simulink model "MotorModel"  (R2021b)
settings: Solver=ode23tb  StartTime=0.0  StopTime=10  RelTol=1e-6
undefined symbols (not defined in the file): sigbuilder_block
libraries: slpidlib x4, aerolibanimutils x1
settings Model: Creator=user  LastModifiedBy=user

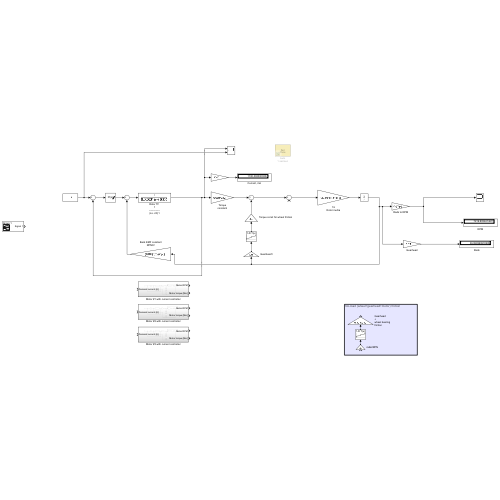
[thumbnail: Simulink's stored preview of the top-level diagram]
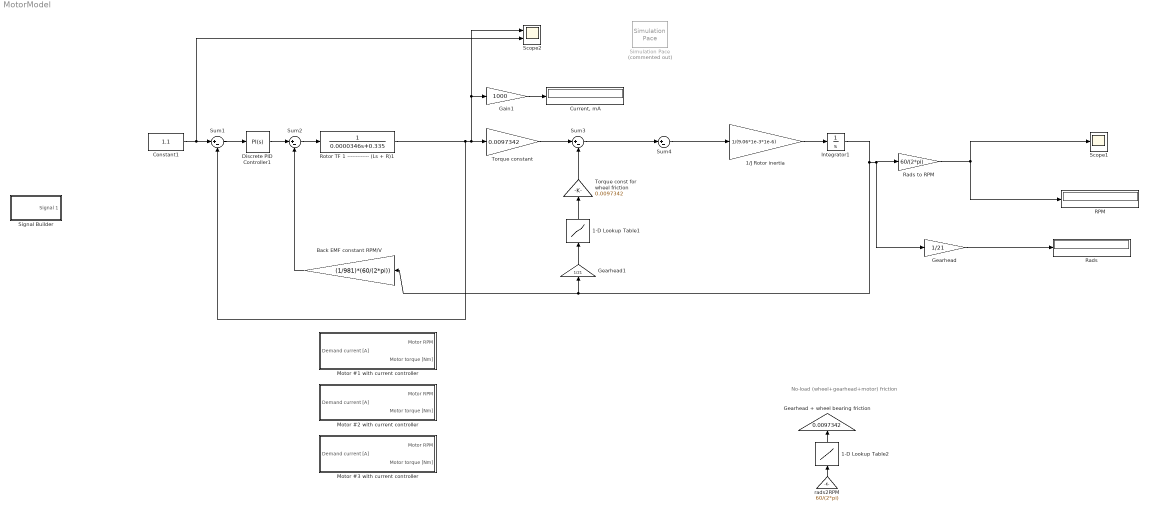
== system MotorModel ==
  note: No-load (wheel+gearhead+motor) friction
  1-D Lookup Table1 : Lookup_n-D  NumberOfTableDimensions=1  BreakpointsForDimension1=[-38 -37 -0.01 0.01 37 38]  Table=[-2 -1.1 -0.5 0.5 1.1 2]  InternalRulePriority=Speed  RndMeth=Simplest  InputSameDT=on
  1-D Lookup Table2 : Lookup_n-D  NumberOfTableDimensions=1  BreakpointsForDimension1=[-10658 -10600 -0.01 0.01 10600 10658]  Table=[-0.5 -0.25 -0.115 0.115 0.25 0.5]  InternalRulePriority=Speed  RndMeth=Simplest  InputSameDT=on
  1/J Rotor inertia : Gain  Gain=1/(9.06*1e-3*1e-6)
  Back EMF constant RPM/V : Gain  Gain=(1/981)*(60/(2*pi))
  Constant1 : Constant  Value=1.1
  "Current, mA" : Display
  Discrete PID Controller1 : slpidlib/PID Controller  Controller=PI  Form=Parallel  TimeDomain=Continuous-time  UseExternalTs=off  SampleTime=1e-6  IntegratorMethod=Forward Euler  FilterMethod=Forward Euler  ControllerParametersSource=internal  P=291  I=291/(1e-6*237)  D=0  UseFilter=on  N=100  TunerSelectOption=Transfer Function Based (PID Tuner App)  InitialConditionSource=internal  InitialConditionForIntegrator=0  InitialConditionForFilter=0  DifferentiatorICPrevScaledInput=0  ExternalReset=none  TrackingMode=off  Kt=1  LimitOutput=on  SatLimitsSource=internal  UpperSaturationLimit=12  LowerSaturationLimit=-12  LinearizeAsGain=off  AntiWindupMode=none  Kb=1  POutMin=[]  POutMax=[]  IOutMin=[]  IOutMax=[]  DOutMin=[]  DOutMax=[]  NOutMin=[]  NOutMax=[]  SumOutMin=[]  SumOutMax=[]  SaturationOutMin=[]  SaturationOutMax=[]  PParamMin=[]  PParamMax=[]  IParamMin=[]  IParamMax=[]  DParamMin=[]  DParamMax=[]  NParamMin=[]  NParamMax=[]  KbParamMin=[]  KbParamMax=[]  KtParamMin=[]  KtParamMax=[]  KbOutMin=[]  KbOutMax=[]  KtOutMin=[]  KtOutMax=[]  IntegratorOutMin=[]  IntegratorOutMax=[]  FilterOutMin=[]  FilterOutMax=[]  SumI1OutMin=[]  SumI1OutMax=[]  SumI2OutMin=[]  SumI2OutMax=[]  SumI3OutMin=[]  SumI3OutMax=[]  SumI4OutMin=[]  SumI4OutMax=[]  SumDOutMin=[]  SumDOutMax=[]  DifferentiatorOutMin=[]  DifferentiatorOutMax=[]  FilterDiffOutCoefMin=[]  FilterDiffOutCoefMax=[]  ReciprocalOutMin=[]  ReciprocalOutMax=[]  SumDenOutMin=[]  SumDenOutMax=[]  SumNumOutMin=[]  SumNumOutMax=[]  DivideOutMin=[]  DivideOutMax=[]  UdiffTsProdOutMin=[]  UdiffTsProdOutMax=[]  NTsProdOutMin=[]  NTsProdOutMax=[]  UintegralTsProdOutMin=[]  UintegralTsProdOutMax=[]  UngainTsProdOutMin=[]  UngainTsProdOutMax=[]  IntegratorContinuousStateAttributes=''  IntegratorStateMustResolveToSignalObject=off  IntegratorRTWStateStorageClass=Auto  FilterContinuousStateAttributes=''  FilterStateMustResolveToSignalObject=off  FilterRTWStateStorageClass=Auto  ParallelPVariant=InternalParameters  IdealPVariant=Disabled  IVariant=InternalParameters  DVariant=Disabled  IntegratorVariant=Continuous  SatVariant=Enabled  AWVariant=Passthrough  PCopyVariant=Disabled  TRVariant=Disabled  FdbkBlocksVariant=Forward  IdealPFdbkVariant=Disabled  SatFdbkVariant=Disabled  DerivativeFilterVariant=Disabled  NVariant=Disabled  NCopyVariant=Disabled_SignalSpec  FilterICVariant=Disabled  IntegratorICVariant=InternalICs  ExternalResetVariant=Disabled  TRSumVariant=Passthrough  SumFdbkVariant=Disabled  SumVariant=Sum_PI  TsampFilterVariant=InternalTs  TsampNgainVariant=Passthrough  TsampIntegralVariant=Passthrough  ExternalSaturationOutDataTypeStr=Inherit: Same as second input
  Gain1 : Gain  Gain=1000
  Gearhead : Gain  Gain=1/21
  Gearhead + wheel bearing friction : Gain  Gain=0.0097342
  Gearhead1 : Gain  Gain=1/21
  Integrator1 : Integrator
  Motor #1 with current controller : Subsystem
  Motor #2 with current controller : Subsystem
  Motor #3 with current controller : Subsystem
  RPM : Display
  Rads : Display
  Rads to RPM : Gain  Gain=60/(2*pi)
  Rotor TF 1 ------------- (Ls + R)1 : TransferFcn  Denominator=[0.0000346 0.335]
  Scope1 : Scope
  Scope2 : Scope  NumInputPorts=2
  Signal Builder : Subsystem  Tag=STV Subsys  LoadFcn=sigbuilder_block('load');  StartFcn=sigbuilder_block('start');  StopFcn=sigbuilder_block('stop');  ClipboardFcn=sigbuilder_block('clipboard');  mask(Sigbuilder block){tuvar=[0:10]}
      mask help: Simulink:masks:SigbuilderBlock_MD
      mask init:
      | if ~strcmp(get_param(bdroot(gcbh),'SimulationStatus'),'stopped') tuvar = sigbuilder_block('maskInit'); end
      settings: CopyFcn=sigbuilder_block('copy');  DeleteFcn=sigbuilder_block('delete');  ModelCloseFcn=sigbuilder_block('modelClose');  PreSaveFcn=sigbuilder_block('preSave');  PauseFcn=sigbuilder_block('pause');  ContinueFcn=sigbuilder_block('continue');  NameChangeFcn=sigbuilder_block('namechange');  OpenFcn=sigbuilder_block('open',[548.25 180.75 550.5 399.75 ]);  CloseFcn=sigbuilder_block('close');
      mask Display: plot(0, 0, 100, 100,[2, 2, 32, 32, 2], [68, 8, 8, 68, 68],[32, 2], [38, 38], [32, 19, 2],[53, 60, 44], [32, 17, 17, 2],[16, 16, 31, 31]);txt = getActiveGroup(gcbh);text(2, 100, txt,'verticalAlignment', 'top');
  Simulation Pace : aerolibanimutils/Simulation Pace  Commented=on  SimulationPace=1  SleepMode=Auto  OutputPaceError=off  SampleTime=1/30
  Sum{1..4} (4 alike) : Sum  Inputs=|+-
  Torque constant : Gain  Gain=0.0097342
  Torque const for wheel friction : Gain  Gain=0.0097342
  rads2RPM : Gain  Gain=60/(2*pi)
  wires:
  Sum3/1 -> Sum4/1
  Gain1/1 -> "Current, mA"/1
  Sum2/1 -> Rotor TF 1 ------------- (Ls + R)1/1
  1/J Rotor inertia/1 -> Integrator1/1
  Sum4/1 -> 1/J Rotor inertia/1
  1-D Lookup Table1/1 -> Torque const for wheel friction/1
  Torque constant/1 -> Sum3/1
  Back EMF constant RPM/V/1 -> Sum2/2
  1-D Lookup Table2/1 -> Gearhead + wheel bearing friction/1
  Sum1/1 -> Discrete PID Controller1/1
  Discrete PID Controller1/1 -> Sum2/1
  Rotor TF 1 ------------- (Ls + R)1/1 -> Sum1/2, Scope2/1, Gain1/1, Torque constant/1
  Constant1/1 -> Scope2/2, Sum1/1
  rads2RPM/1 -> 1-D Lookup Table2/1
  Torque const for wheel friction/1 -> Sum3/2
  Gearhead/1 -> Rads/1
  Gearhead1/1 -> 1-D Lookup Table1/1
  Integrator1/1 -> Gearhead1/1, Back EMF constant RPM/V/1, Gearhead/1, Rads to RPM/1
  Rads to RPM/1 -> RPM/1, Scope1/1

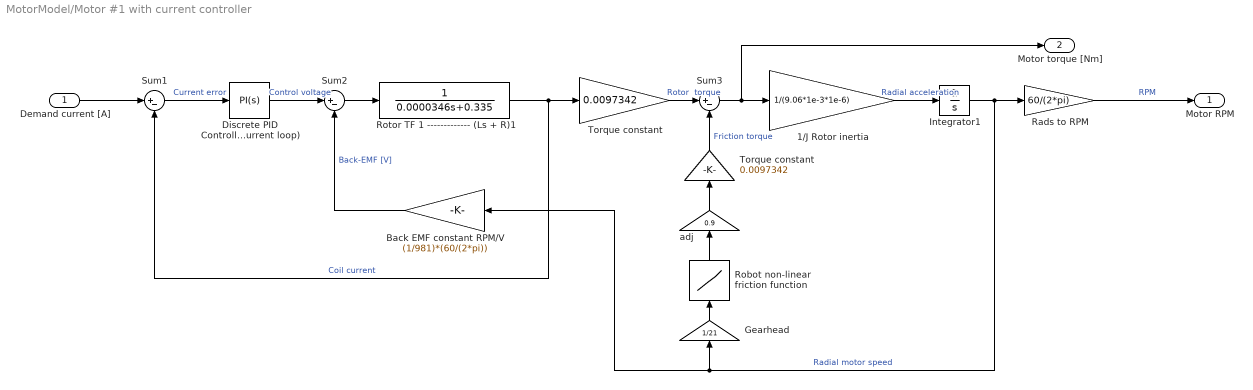
== system MotorModel/Motor #1 with current controller ==
  Demand current [A] : Inport
  1/J Rotor inertia : Gain  Gain=1/(9.06*1e-3*1e-6)
  Back EMF constant RPM/V : Gain  Gain=(1/981)*(60/(2*pi))
  Discrete PID Controller (current loop) : slpidlib/PID Controller  Controller=PI  Form=Parallel  TimeDomain=Continuous-time  UseExternalTs=off  SampleTime=1e-6  IntegratorMethod=Forward Euler  FilterMethod=Forward Euler  ControllerParametersSource=internal  P=291  I=291/(1e-6*237)  D=0  UseFilter=on  N=100  TunerSelectOption=Transfer Function Based (PID Tuner App)  InitialConditionSource=internal  InitialConditionForIntegrator=0  InitialConditionForFilter=0  DifferentiatorICPrevScaledInput=0  ExternalReset=none  TrackingMode=off  Kt=1  LimitOutput=on  SatLimitsSource=internal  UpperSaturationLimit=12  LowerSaturationLimit=-12  LinearizeAsGain=off  AntiWindupMode=none  Kb=1  POutMin=[]  POutMax=[]  IOutMin=[]  IOutMax=[]  DOutMin=[]  DOutMax=[]  NOutMin=[]  NOutMax=[]  SumOutMin=[]  SumOutMax=[]  SaturationOutMin=[]  SaturationOutMax=[]  PParamMin=[]  PParamMax=[]  IParamMin=[]  IParamMax=[]  DParamMin=[]  DParamMax=[]  NParamMin=[]  NParamMax=[]  KbParamMin=[]  KbParamMax=[]  KtParamMin=[]  KtParamMax=[]  KbOutMin=[]  KbOutMax=[]  KtOutMin=[]  KtOutMax=[]  IntegratorOutMin=[]  IntegratorOutMax=[]  FilterOutMin=[]  FilterOutMax=[]  SumI1OutMin=[]  SumI1OutMax=[]  SumI2OutMin=[]  SumI2OutMax=[]  SumI3OutMin=[]  SumI3OutMax=[]  SumI4OutMin=[]  SumI4OutMax=[]  SumDOutMin=[]  SumDOutMax=[]  DifferentiatorOutMin=[]  DifferentiatorOutMax=[]  FilterDiffOutCoefMin=[]  FilterDiffOutCoefMax=[]  ReciprocalOutMin=[]  ReciprocalOutMax=[]  SumDenOutMin=[]  SumDenOutMax=[]  SumNumOutMin=[]  SumNumOutMax=[]  DivideOutMin=[]  DivideOutMax=[]  UdiffTsProdOutMin=[]  UdiffTsProdOutMax=[]  NTsProdOutMin=[]  NTsProdOutMax=[]  UintegralTsProdOutMin=[]  UintegralTsProdOutMax=[]  UngainTsProdOutMin=[]  UngainTsProdOutMax=[]  IntegratorContinuousStateAttributes=''  IntegratorStateMustResolveToSignalObject=off  IntegratorRTWStateStorageClass=Auto  FilterContinuousStateAttributes=''  FilterStateMustResolveToSignalObject=off  FilterRTWStateStorageClass=Auto  ParallelPVariant=InternalParameters  IdealPVariant=Disabled  IVariant=InternalParameters  DVariant=Disabled  IntegratorVariant=Continuous  SatVariant=Enabled  AWVariant=Passthrough  PCopyVariant=Disabled  TRVariant=Disabled  FdbkBlocksVariant=Forward  IdealPFdbkVariant=Disabled  SatFdbkVariant=Disabled  DerivativeFilterVariant=Disabled  NVariant=Disabled  NCopyVariant=Disabled_SignalSpec  FilterICVariant=Disabled  IntegratorICVariant=InternalICs  ExternalResetVariant=Disabled  TRSumVariant=Passthrough  SumFdbkVariant=Disabled  SumVariant=Sum_PI  TsampFilterVariant=InternalTs  TsampNgainVariant=Passthrough  TsampIntegralVariant=Passthrough  ExternalSaturationOutDataTypeStr=Inherit: Same as second input
  "Gearhead " : Gain  Gain=1/21
  Integrator1 : Integrator
  Rads to RPM : Gain  Gain=60/(2*pi)
  Robot non-linear friction function : Lookup_n-D  NumberOfTableDimensions=1  BreakpointsForDimension1=[-38 -37 -0.01 0.01 37 38]  Table=[-2 -1.1 -0.5 0.5 1.1 2]  InternalRulePriority=Speed  RndMeth=Simplest  InputSameDT=on
  Rotor TF 1 ------------- (Ls + R)1 : TransferFcn  Denominator=[0.0000346 0.335]
  Sum1 : Sum  Inputs=|+-
  Sum2 : Sum  Inputs=|+-
  Sum3 : Sum  Inputs=|+-
  Torque constant : Gain  Gain=0.0097342
  "Torque constant " : Gain  Gain=0.0097342
  adj : Gain  Gain=0.9
  Motor RPM : Outport
  Motor torque [Nm] : Outport  Port=2
  wires:
  Discrete PID Controller (current loop)/1 -> Sum2/1  "Control voltage"
  Sum1/1 -> Discrete PID Controller (current loop)/1  "Current error"
  Rotor TF 1 ------------- (Ls + R)1/1 -> Torque constant/1, Sum1/2  "Coil current"
  Back EMF constant RPM/V/1 -> Sum2/2  "Back-EMF [V]"
  Sum2/1 -> Rotor TF 1 ------------- (Ls + R)1/1
  Torque constant/1 -> Sum3/1  "Rotor  torque"
  Robot non-linear friction function/1 -> adj/1
  Sum3/1 -> Motor torque [Nm]/1, 1/J Rotor inertia/1
  "Gearhead "/1 -> Robot non-linear friction function/1
  1/J Rotor inertia/1 -> Integrator1/1  "Radial acceleration"
  Integrator1/1 -> Rads to RPM/1, "Gearhead "/1, Back EMF constant RPM/V/1  "Radial motor speed"
  "Torque constant "/1 -> Sum3/2  "Friction torque"
  Demand current [A]/1 -> Sum1/1
  Rads to RPM/1 -> Motor RPM/1  "RPM"
  adj/1 -> "Torque constant "/1

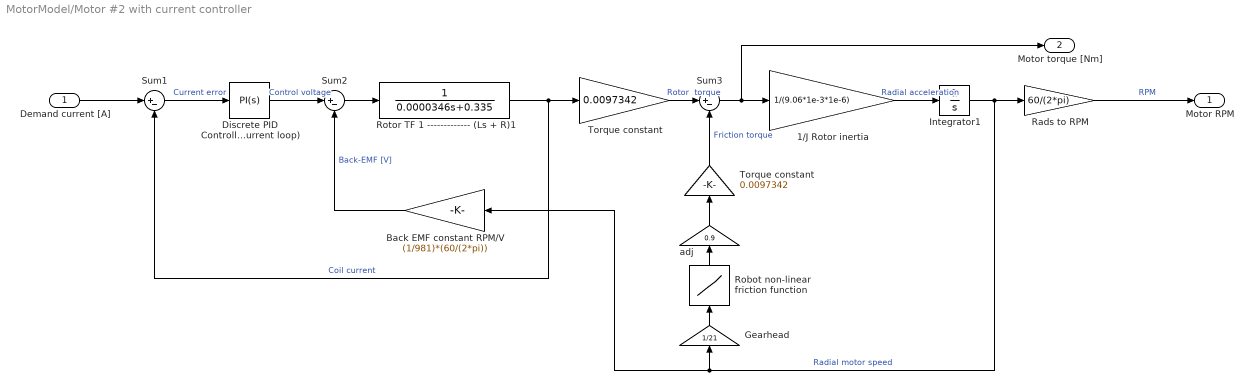
== system MotorModel/Motor #2 with current controller ==
  Demand current [A] : Inport
  1/J Rotor inertia : Gain  Gain=1/(9.06*1e-3*1e-6)
  Back EMF constant RPM/V : Gain  Gain=(1/981)*(60/(2*pi))
  Discrete PID Controller (current loop) : slpidlib/PID Controller  Controller=PI  Form=Parallel  TimeDomain=Continuous-time  UseExternalTs=off  SampleTime=1e-6  IntegratorMethod=Forward Euler  FilterMethod=Forward Euler  ControllerParametersSource=internal  P=291  I=291/(1e-6*237)  D=0  UseFilter=on  N=100  TunerSelectOption=Transfer Function Based (PID Tuner App)  InitialConditionSource=internal  InitialConditionForIntegrator=0  InitialConditionForFilter=0  DifferentiatorICPrevScaledInput=0  ExternalReset=none  TrackingMode=off  Kt=1  LimitOutput=on  SatLimitsSource=internal  UpperSaturationLimit=12  LowerSaturationLimit=-12  LinearizeAsGain=off  AntiWindupMode=none  Kb=1  POutMin=[]  POutMax=[]  IOutMin=[]  IOutMax=[]  DOutMin=[]  DOutMax=[]  NOutMin=[]  NOutMax=[]  SumOutMin=[]  SumOutMax=[]  SaturationOutMin=[]  SaturationOutMax=[]  PParamMin=[]  PParamMax=[]  IParamMin=[]  IParamMax=[]  DParamMin=[]  DParamMax=[]  NParamMin=[]  NParamMax=[]  KbParamMin=[]  KbParamMax=[]  KtParamMin=[]  KtParamMax=[]  KbOutMin=[]  KbOutMax=[]  KtOutMin=[]  KtOutMax=[]  IntegratorOutMin=[]  IntegratorOutMax=[]  FilterOutMin=[]  FilterOutMax=[]  SumI1OutMin=[]  SumI1OutMax=[]  SumI2OutMin=[]  SumI2OutMax=[]  SumI3OutMin=[]  SumI3OutMax=[]  SumI4OutMin=[]  SumI4OutMax=[]  SumDOutMin=[]  SumDOutMax=[]  DifferentiatorOutMin=[]  DifferentiatorOutMax=[]  FilterDiffOutCoefMin=[]  FilterDiffOutCoefMax=[]  ReciprocalOutMin=[]  ReciprocalOutMax=[]  SumDenOutMin=[]  SumDenOutMax=[]  SumNumOutMin=[]  SumNumOutMax=[]  DivideOutMin=[]  DivideOutMax=[]  UdiffTsProdOutMin=[]  UdiffTsProdOutMax=[]  NTsProdOutMin=[]  NTsProdOutMax=[]  UintegralTsProdOutMin=[]  UintegralTsProdOutMax=[]  UngainTsProdOutMin=[]  UngainTsProdOutMax=[]  IntegratorContinuousStateAttributes=''  IntegratorStateMustResolveToSignalObject=off  IntegratorRTWStateStorageClass=Auto  FilterContinuousStateAttributes=''  FilterStateMustResolveToSignalObject=off  FilterRTWStateStorageClass=Auto  ParallelPVariant=InternalParameters  IdealPVariant=Disabled  IVariant=InternalParameters  DVariant=Disabled  IntegratorVariant=Continuous  SatVariant=Enabled  AWVariant=Passthrough  PCopyVariant=Disabled  TRVariant=Disabled  FdbkBlocksVariant=Forward  IdealPFdbkVariant=Disabled  SatFdbkVariant=Disabled  DerivativeFilterVariant=Disabled  NVariant=Disabled  NCopyVariant=Disabled_SignalSpec  FilterICVariant=Disabled  IntegratorICVariant=InternalICs  ExternalResetVariant=Disabled  TRSumVariant=Passthrough  SumFdbkVariant=Disabled  SumVariant=Sum_PI  TsampFilterVariant=InternalTs  TsampNgainVariant=Passthrough  TsampIntegralVariant=Passthrough  ExternalSaturationOutDataTypeStr=Inherit: Same as second input
  "Gearhead " : Gain  Gain=1/21
  Integrator1 : Integrator
  Rads to RPM : Gain  Gain=60/(2*pi)
  Robot non-linear friction function : Lookup_n-D  NumberOfTableDimensions=1  BreakpointsForDimension1=[-38 -37 -0.01 0.01 37 38]  Table=[-2 -1.1 -0.5 0.5 1.1 2]  InternalRulePriority=Speed  RndMeth=Simplest  InputSameDT=on
  Rotor TF 1 ------------- (Ls + R)1 : TransferFcn  Denominator=[0.0000346 0.335]
  Sum1 : Sum  Inputs=|+-
  Sum2 : Sum  Inputs=|+-
  Sum3 : Sum  Inputs=|+-
  Torque constant : Gain  Gain=0.0097342
  "Torque constant " : Gain  Gain=0.0097342
  adj : Gain  Gain=0.9
  Motor RPM : Outport
  Motor torque [Nm] : Outport  Port=2
  wires:
  Rads to RPM/1 -> Motor RPM/1  "RPM"
  Demand current [A]/1 -> Sum1/1
  "Torque constant "/1 -> Sum3/2  "Friction torque"
  Integrator1/1 -> Back EMF constant RPM/V/1, "Gearhead "/1, Rads to RPM/1  "Radial motor speed"
  1/J Rotor inertia/1 -> Integrator1/1  "Radial acceleration"
  "Gearhead "/1 -> Robot non-linear friction function/1
  Sum3/1 -> 1/J Rotor inertia/1, Motor torque [Nm]/1
  Robot non-linear friction function/1 -> adj/1
  Torque constant/1 -> Sum3/1  "Rotor  torque"
  Sum2/1 -> Rotor TF 1 ------------- (Ls + R)1/1
  Back EMF constant RPM/V/1 -> Sum2/2  "Back-EMF [V]"
  Rotor TF 1 ------------- (Ls + R)1/1 -> Sum1/2, Torque constant/1  "Coil current"
  Sum1/1 -> Discrete PID Controller (current loop)/1  "Current error"
  Discrete PID Controller (current loop)/1 -> Sum2/1  "Control voltage"
  adj/1 -> "Torque constant "/1

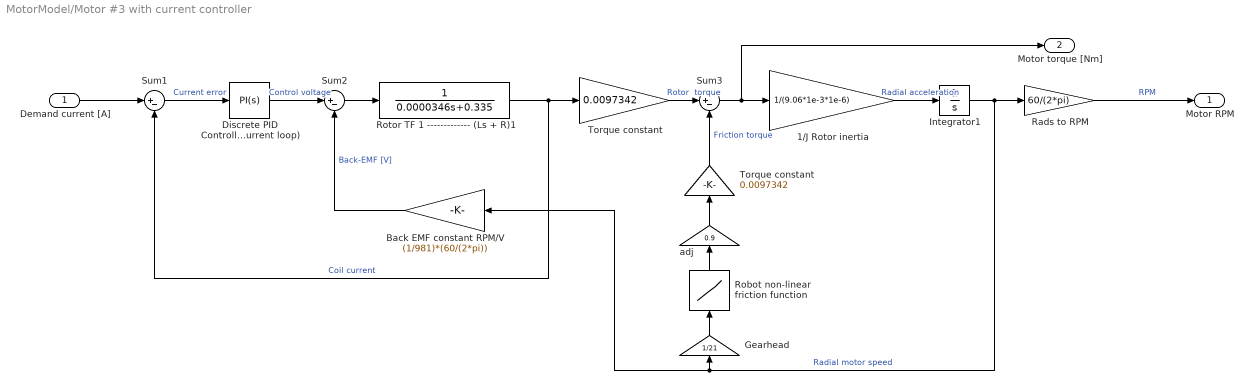
== system MotorModel/Motor #3 with current controller ==
  Demand current [A] : Inport
  1/J Rotor inertia : Gain  Gain=1/(9.06*1e-3*1e-6)
  Back EMF constant RPM/V : Gain  Gain=(1/981)*(60/(2*pi))
  Discrete PID Controller (current loop) : slpidlib/PID Controller  Controller=PI  Form=Parallel  TimeDomain=Continuous-time  UseExternalTs=off  SampleTime=1e-6  IntegratorMethod=Forward Euler  FilterMethod=Forward Euler  ControllerParametersSource=internal  P=291  I=291/(1e-6*237)  D=0  UseFilter=on  N=100  TunerSelectOption=Transfer Function Based (PID Tuner App)  InitialConditionSource=internal  InitialConditionForIntegrator=0  InitialConditionForFilter=0  DifferentiatorICPrevScaledInput=0  ExternalReset=none  TrackingMode=off  Kt=1  LimitOutput=on  SatLimitsSource=internal  UpperSaturationLimit=12  LowerSaturationLimit=-12  LinearizeAsGain=off  AntiWindupMode=none  Kb=1  POutMin=[]  POutMax=[]  IOutMin=[]  IOutMax=[]  DOutMin=[]  DOutMax=[]  NOutMin=[]  NOutMax=[]  SumOutMin=[]  SumOutMax=[]  SaturationOutMin=[]  SaturationOutMax=[]  PParamMin=[]  PParamMax=[]  IParamMin=[]  IParamMax=[]  DParamMin=[]  DParamMax=[]  NParamMin=[]  NParamMax=[]  KbParamMin=[]  KbParamMax=[]  KtParamMin=[]  KtParamMax=[]  KbOutMin=[]  KbOutMax=[]  KtOutMin=[]  KtOutMax=[]  IntegratorOutMin=[]  IntegratorOutMax=[]  FilterOutMin=[]  FilterOutMax=[]  SumI1OutMin=[]  SumI1OutMax=[]  SumI2OutMin=[]  SumI2OutMax=[]  SumI3OutMin=[]  SumI3OutMax=[]  SumI4OutMin=[]  SumI4OutMax=[]  SumDOutMin=[]  SumDOutMax=[]  DifferentiatorOutMin=[]  DifferentiatorOutMax=[]  FilterDiffOutCoefMin=[]  FilterDiffOutCoefMax=[]  ReciprocalOutMin=[]  ReciprocalOutMax=[]  SumDenOutMin=[]  SumDenOutMax=[]  SumNumOutMin=[]  SumNumOutMax=[]  DivideOutMin=[]  DivideOutMax=[]  UdiffTsProdOutMin=[]  UdiffTsProdOutMax=[]  NTsProdOutMin=[]  NTsProdOutMax=[]  UintegralTsProdOutMin=[]  UintegralTsProdOutMax=[]  UngainTsProdOutMin=[]  UngainTsProdOutMax=[]  IntegratorContinuousStateAttributes=''  IntegratorStateMustResolveToSignalObject=off  IntegratorRTWStateStorageClass=Auto  FilterContinuousStateAttributes=''  FilterStateMustResolveToSignalObject=off  FilterRTWStateStorageClass=Auto  ParallelPVariant=InternalParameters  IdealPVariant=Disabled  IVariant=InternalParameters  DVariant=Disabled  IntegratorVariant=Continuous  SatVariant=Enabled  AWVariant=Passthrough  PCopyVariant=Disabled  TRVariant=Disabled  FdbkBlocksVariant=Forward  IdealPFdbkVariant=Disabled  SatFdbkVariant=Disabled  DerivativeFilterVariant=Disabled  NVariant=Disabled  NCopyVariant=Disabled_SignalSpec  FilterICVariant=Disabled  IntegratorICVariant=InternalICs  ExternalResetVariant=Disabled  TRSumVariant=Passthrough  SumFdbkVariant=Disabled  SumVariant=Sum_PI  TsampFilterVariant=InternalTs  TsampNgainVariant=Passthrough  TsampIntegralVariant=Passthrough  ExternalSaturationOutDataTypeStr=Inherit: Same as second input
  "Gearhead " : Gain  Gain=1/21
  Integrator1 : Integrator
  Rads to RPM : Gain  Gain=60/(2*pi)
  Robot non-linear friction function : Lookup_n-D  NumberOfTableDimensions=1  BreakpointsForDimension1=[-38 -37 -0.01 0.01 37 38]  Table=[-2 -1.2 -0.55 0.55 1.2 2]  InternalRulePriority=Speed  RndMeth=Simplest  InputSameDT=on
  Rotor TF 1 ------------- (Ls + R)1 : TransferFcn  Denominator=[0.0000346 0.335]
  Sum1 : Sum  Inputs=|+-
  Sum2 : Sum  Inputs=|+-
  Sum3 : Sum  Inputs=|+-
  Torque constant : Gain  Gain=0.0097342
  "Torque constant " : Gain  Gain=0.0097342
  adj : Gain  Gain=0.9
  Motor RPM : Outport
  Motor torque [Nm] : Outport  Port=2
  wires:
  Discrete PID Controller (current loop)/1 -> Sum2/1  "Control voltage"
  Sum1/1 -> Discrete PID Controller (current loop)/1  "Current error"
  Rotor TF 1 ------------- (Ls + R)1/1 -> Torque constant/1, Sum1/2  "Coil current"
  Back EMF constant RPM/V/1 -> Sum2/2  "Back-EMF [V]"
  Sum2/1 -> Rotor TF 1 ------------- (Ls + R)1/1
  Torque constant/1 -> Sum3/1  "Rotor  torque"
  Robot non-linear friction function/1 -> adj/1
  Sum3/1 -> Motor torque [Nm]/1, 1/J Rotor inertia/1
  1/J Rotor inertia/1 -> Integrator1/1  "Radial acceleration"
  Integrator1/1 -> Rads to RPM/1, "Gearhead "/1, Back EMF constant RPM/V/1  "Radial motor speed"
  "Torque constant "/1 -> Sum3/2  "Friction torque"
  Demand current [A]/1 -> Sum1/1
  Rads to RPM/1 -> Motor RPM/1  "RPM"
  "Gearhead "/1 -> Robot non-linear friction function/1
  adj/1 -> "Torque constant "/1

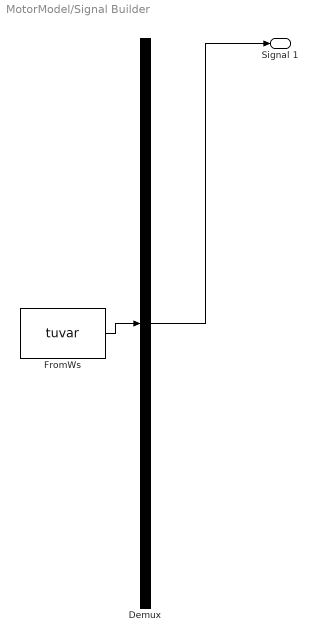
== system MotorModel/Signal Builder ==
  Demux : Demux  Tag=STV Demux  Outputs=1
      settings: DisplayOption=none
  FromWs : FromWorkspace  Tag=STV FromWs  VariableName=tuvar
      SigBuilderData=|
      | common.afterFinalStr = 'Extrapolate'
      | common.sampleTime = 0
      | dataSet.timeRange = [0 0.25]
      | dataSet.name = 'Group 1'
      | sbobj.Groups.Name = 'Group 1'
      | sbobj.Groups.Signals.Name = 'Signal 1'
      | sbobj.Groups.Signals.XData = [0 0.05 0.05 0.075 0.075 0.125 0.125 0.15 0.15 0.25]
      | sbobj.Groups.Signals.YData = [0 0 1 1 -1 -1 1 1 0 0]
      | sbobj.Groups.TimeRange = [0 0.25]
  Signal 1 : Outport  Tag=STV Outport
  wires:
  Demux/1 -> Signal 1/1
  FromWs/1 -> Demux/1
